simulink model "circuit3Diz"  (Simulink 5.0)
settings: Solver=ode23tb  StartTime=0.0  StopTime=0.1  FixedStep=25e-6  RelTol=1e-4
undefined symbols (not defined in the file): T
libraries: powerlib2 x11
settings Model: LastModifiedBy=Администратор

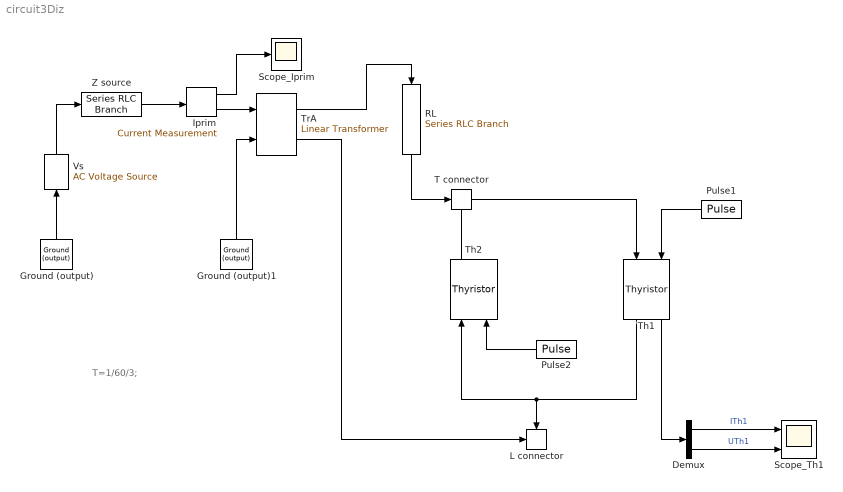
== system circuit3Diz ==
  note: T=1/60/3;
  Demux : Demux  Outputs=2
  Ground (output) : powerlib2/Connectors/Ground (output)  Tag=PoWeRsYsTeMbLoCk  Orientation=up  PSBOutputType=1
  Ground (output)1 : powerlib2/Connectors/Ground (output)  Tag=PoWeRsYsTeMbLoCk  Orientation=up  PSBOutputType=1
  Iprim : powerlib2/Measurements/Current Measurement  Tag=PoWeRsYsTeMmEaSuReMeNt  PhasorSimulation=off  OutputType=Magnitude  PSBOutputType=01  PSBequivalent=1
  L connector : powerlib2/Connectors/L connector  Tag=PoWeRsYsTeMbLoCk
  Pulse1 : DiscretePulseGenerator  Orientation=left  PulseType=Time based  Period=1.66666666666666666666666666666e-2  PhaseDelay=1.66666666666666666666666666666e-2+T
  Pulse2 : DiscretePulseGenerator  Orientation=left  PulseType=Time based  Period=1.66666666666666666666666666666e-2  PhaseDelay=0.025+T
  RL : powerlib2/Elements/Series RLC Branch  Tag=PoWeRsYsTeMbLoCk  Orientation=down  a=70.5e-3  b=18.7e-03  c=inf  mesure=None  PSBOutputType=1
  "Scope_Iprim " : Scope
  Scope_Th1 : Scope  NumInputPorts=2
      settings: YMin=-5~-5  YMax=5~5
  T connector : powerlib2/Connectors/T connector  Tag=PoWeRsYsTeMbLoCk  PSBOutputType=1
  Th1 : powerlib2/Power Electronics/Thyristor  Tag=PoWeRsYsTeMbLoCk  Orientation=down  Ron=1e-03  Lon=0  Vf=11.2  IC=0  Rs=500  Cs=0.15e-6  PSBOutputType=10
  Th2 : powerlib2/Power Electronics/Thyristor  Tag=PoWeRsYsTeMbLoCk  Orientation=up  Ron=1e-03  Lon=0  Vf=11.2  IC=0  Rs=inf  Cs=0  PSBOutputType=10
  TrA : powerlib2/Elements/Linear Transformer  Tag=PoWeRsYsTeMbLoCk  a=[110e6 60]  b=[424.4e3 0.002 0.15]  c=[16e3 0.002 0]  w3check=off  d=[60e3 0.005 0.02]  e=[500 500]  mesure=None  PSBOutputType=1111
  Vs : powerlib2/Electrical Sources/AC Voltage Source  Tag=PoWeRsYsTeMbLoCk  Description=source block  Orientation=up  A=600192.2358711415387114366945546  P=0  F=60  stime=0  mesure=None  PSBOutputType=1
  Z source : powerlib2/Elements/Series RLC Branch  Tag=PoWeRsYsTeMbLoCk  a=2.7  b=71.65e-03  c=inf  mesure=None  PSBOutputType=1
  wires:
  Th1/1 -> Th2/1, L connector/Enable
  Th2/1 -> T connector/Enable
  T connector/1 -> Th1/1
  Vs/1 -> Z source/1
  Z source/1 -> Iprim/1
  Iprim/2 -> TrA/1
  Iprim/1 -> "Scope_Iprim "/1
  RL/1 -> T connector/1
  TrA/1 -> RL/1
  TrA/2 -> L connector/1
  Ground (output)/1 -> Vs/1
  Ground (output)1/1 -> TrA/2
  Th1/2 -> Demux/1
  Demux/1 -> Scope_Th1/1  "ITh1"
  Demux/2 -> Scope_Th1/2  "UTh1"
  Pulse1/1 -> Th1/2
  Pulse2/1 -> Th2/2
